simulink model "CrazyClover_thrust_angular_vel_control1"  (R2020b)
settings: Solver=VariableStepAuto  StartTime=0.0  StopTime=1.5  RelTol=1e-3
values from neighbouring files (symbols this model uses):
  controller_matrix = [mass/(4*gravity)*1000 mass/(4*gravity)*1000 mass/(4*gravity)*1000 mass/(4*gravity)*1000 ... (first row only)    [sim_param.m]
  kM1 = Armlength /sqrt(2)    [sim_param.m]
  kM2 = Armlength /sqrt(2)    [sim_param.m]
  kM3 = 1    [sim_param.m]
undefined symbols (not defined in the file or in its folder): Pitchrate, Rollrate, Yawrate
libraries: pid_lib x6
settings Model: Creator=kt012  LastModifiedBy=kt012

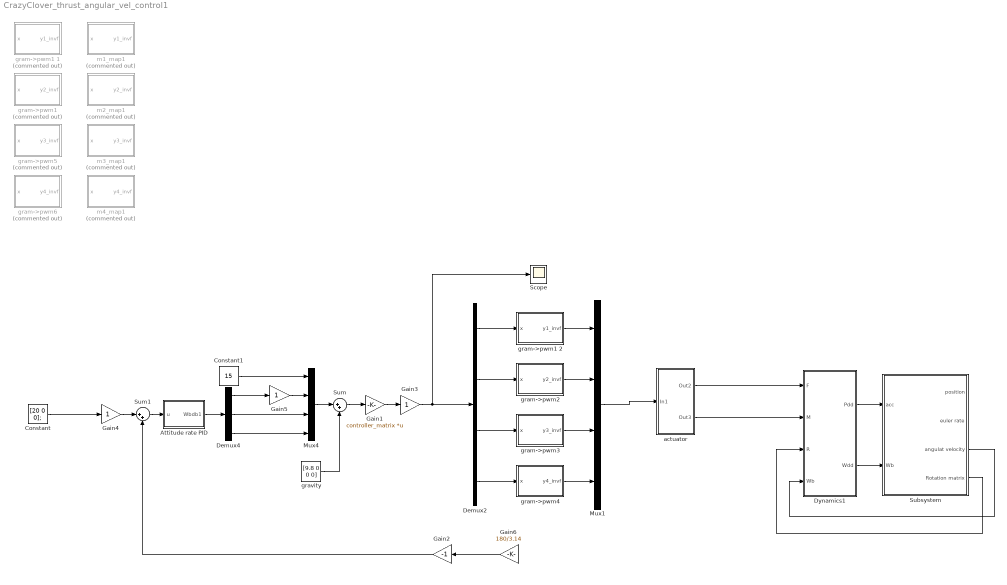
== system CrazyClover_thrust_angular_vel_control1 ==
  Attitude rate PID : Subsystem
  Constant : Constant  Value=[20 0 0];
  Constant1 : Constant  Value=15
  Demux2 : Demux
  Demux4 : Demux  Outputs=3
  Dynamics1 : MATLAB Function  TreatAsAtomicUnit=on
  Gain1 : Gain  Gain=controller_matrix  Multiplication=Matrix(K*u)
  Gain2 : Gain  Gain=-1
  Gain3 : Gain
  Gain4 : Gain
  Gain5 : Gain
  Gain6 : Gain  Gain=180/3.14
  Mux1 : Mux
  Mux4 : Mux
  Scope : Scope
  Subsystem : Subsystem
  Sum : Sum  Inputs=|++
  Sum1 : Sum  Inputs=|++
  actuator : Subsystem
  gram->pwm1 : MATLAB Function  Commented=on  TreatAsAtomicUnit=on
  gram->pwm1 1 : MATLAB Function  Commented=on  TreatAsAtomicUnit=on
  gram->pwm1 2 : MATLAB Function  TreatAsAtomicUnit=on
  gram->pwm2 : MATLAB Function  TreatAsAtomicUnit=on
  gram->pwm3 : MATLAB Function  TreatAsAtomicUnit=on
  gram->pwm4 : MATLAB Function  TreatAsAtomicUnit=on
  gram->pwm5 : MATLAB Function  Commented=on  TreatAsAtomicUnit=on
  gram->pwm6 : MATLAB Function  Commented=on  TreatAsAtomicUnit=on
  gravity : Constant  Value=[9.8 0 0 0]
  m1_map1 : MATLAB Function  Commented=on  TreatAsAtomicUnit=on
  m2_map1 : MATLAB Function  Commented=on  TreatAsAtomicUnit=on
  m3_map1 : MATLAB Function  Commented=on  TreatAsAtomicUnit=on
  m4_map1 : MATLAB Function  Commented=on  TreatAsAtomicUnit=on
  wires:
  Gain1/1 -> Gain3/1
  Gain3/1 -> Scope/1, Demux2/1
  Demux2/1 -> gram->pwm1 2/1(x)
  Demux2/2 -> gram->pwm2/1(x)
  Demux2/3 -> gram->pwm3/1(x)
  Demux2/4 -> gram->pwm4/1(x)
  gravity/1 -> Sum/2
  Sum/1 -> Gain1/1
  Attitude rate PID/1(Wbdb1) -> Demux4/1
  Gain2/1 -> Sum1/2
  Demux4/1 -> Gain5/1
  Demux4/3 -> Mux4/4
  Constant1/1 -> Mux4/1
  Mux4/1 -> Sum/1
  Demux4/2 -> Mux4/3
  Gain5/1 -> Mux4/2
  Sum1/1 -> Attitude rate PID/1(u)
  Constant/1 -> Gain4/1
  Gain4/1 -> Sum1/1
  Gain6/1 -> Gain2/1
  gram->pwm1 2/1(y1_invf) -> Mux1/1
  gram->pwm2/1(y2_invf) -> Mux1/2
  gram->pwm3/1(y3_invf) -> Mux1/3
  gram->pwm4/1(y4_invf) -> Mux1/4
  Dynamics1/1(Pdd) -> Subsystem/1(acc)
  Dynamics1/2(Wdd) -> Subsystem/2(Wb)
  Subsystem/3(angulat velocity) -> Dynamics1/4(Wb)
  Subsystem/4(Rotation matrix) -> Dynamics1/3(R)
  Mux1/1 -> actuator/1(In1)
  actuator/1(Out2) -> Dynamics1/1(F)
  actuator/2(Out3) -> Dynamics1/2(M)

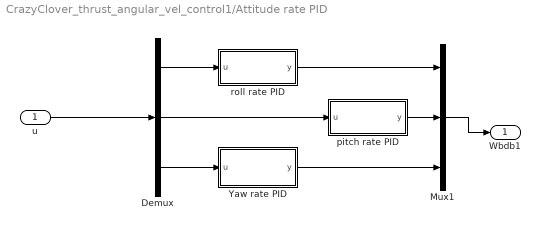
== system CrazyClover_thrust_angular_vel_control1/Attitude rate PID ==
  u : Inport
  Demux : Demux  Outputs=3
  Mux1 : Mux  Inputs=3
  "Yaw rate PID " : Subsystem
  pitch rate PID : Subsystem
  "roll rate PID " : Subsystem
  Wbdb1 : Outport
  wires:
  "roll rate PID "/1(y) -> Mux1/1
  pitch rate PID/1(y) -> Mux1/2
  Demux/2 -> pitch rate PID/1(u)
  u/1 -> Demux/1
  Demux/3 -> "Yaw rate PID "/1(u)
  Demux/1 -> "roll rate PID "/1(u)
  "Yaw rate PID "/1(y) -> Mux1/3
  Mux1/1 -> Wbdb1/1

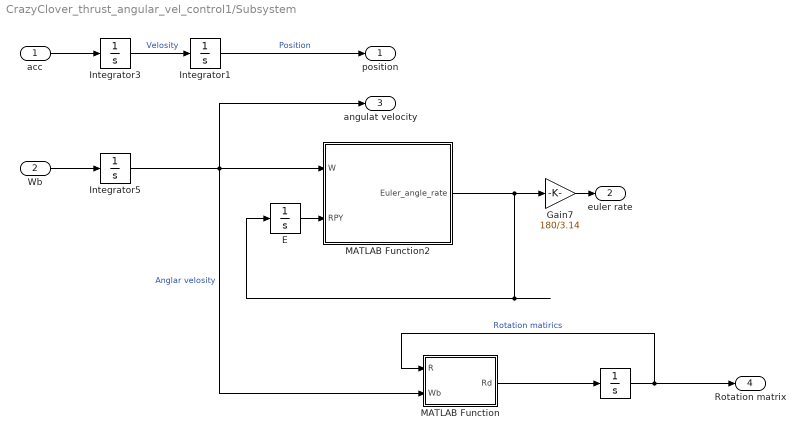
== system CrazyClover_thrust_angular_vel_control1/Subsystem ==
  acc : Inport
  Wb : Inport  Port=2
  " " : Integrator  InitialCondition=[1 0 0; 0 1 0; 0 0 1];  ContinuousStateAttributes="\"\""
  E : Integrator  InitialCondition=[0 0 0];
  Gain7 : Gain  Gain=180/3.14
  Integrator1 : Integrator  InitialCondition=[0 0 0];
  Integrator3 : Integrator  InitialCondition=[0 0 0];
  Integrator5 : Integrator  InitialCondition=[0 0 0];
  MATLAB Function : MATLAB Function  TreatAsAtomicUnit=on
  MATLAB Function2 : MATLAB Function  TreatAsAtomicUnit=on
  position : Outport
  euler rate : Outport  Port=2
  angulat velocity : Outport  Port=3
  Rotation matrix : Outport  Port=4
  wires:
  MATLAB Function2/1(Euler_angle_rate) -> E/1, Gain7/1
  acc/1 -> Integrator3/1
  Integrator1/1 -> position/1  "Position"
  Integrator3/1 -> Integrator1/1  "Velosity"
  E/1 -> MATLAB Function2/2(RPY)
  Wb/1 -> Integrator5/1
  Gain7/1 -> euler rate/1
  MATLAB Function/1(Rd) -> " "/1
  Integrator5/1 -> MATLAB Function/2(Wb), angulat velocity/1, MATLAB Function2/1(W)  "Anglar velosity"
  " "/1 -> Rotation matrix/1, MATLAB Function/1(R)  "Rotation matirics"

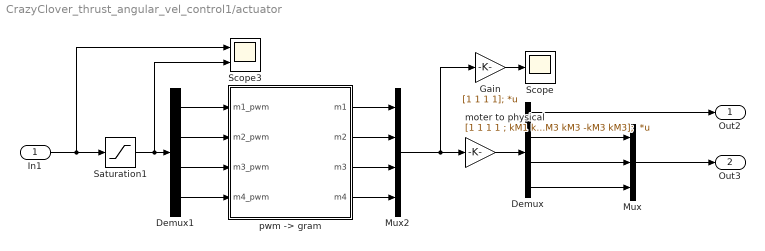
== system CrazyClover_thrust_angular_vel_control1/actuator ==
  In1 : Inport
  Demux : Demux
  Demux1 : Demux
  Gain : Gain  Gain=[1 1 1 1];  Multiplication=Matrix(K*u)
  Mux : Mux  Inputs=3
  Mux2 : Mux
  Saturation1 : Saturate  UpperLimit=40000  LowerLimit=0
  Scope : Scope
  Scope3 : Scope  NumInputPorts=2
  moter to physical : Gain  Gain=[1 1 1 1 ; kM1 kM1 -kM1 -kM1; -kM2 kM2 kM2 -kM2; -kM3 kM3 -kM3 kM3];  Multiplication=Matrix(K*u)
  "pwm -> gram" : MATLAB Function  TreatAsAtomicUnit=on
  Out2 : Outport
  Out3 : Outport  Port=2
  wires:
  Demux/2 -> Mux/1
  "pwm -> gram"/3(m3) -> Mux2/3
  Demux1/2 -> "pwm -> gram"/2(m2_pwm)
  Demux/4 -> Mux/3
  Demux/3 -> Mux/2
  moter to physical/1 -> Demux/1
  "pwm -> gram"/1(m1) -> Mux2/1
  Mux2/1 -> Gain/1, moter to physical/1
  Gain/1 -> Scope/1
  Saturation1/1 -> Scope3/2, Demux1/1
  In1/1 -> Scope3/1, Saturation1/1
  Demux1/3 -> "pwm -> gram"/3(m3_pwm)
  "pwm -> gram"/4(m4) -> Mux2/4
  "pwm -> gram"/2(m2) -> Mux2/2
  Demux1/4 -> "pwm -> gram"/4(m4_pwm)
  Demux1/1 -> "pwm -> gram"/1(m1_pwm)
  Mux/1 -> Out3/1
  Demux/1 -> Out2/1

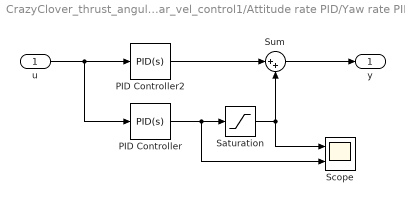
== system CrazyClover_thrust_angular_vel_control1/Attitude rate PID/Yaw rate PID  ==
  u : Inport
  PID Controller : pid_lib/PID Controller  Controller=PID  Form=Parallel  TimeDomain=Continuous-time  UseExternalTs=off  SampleTime=-1  IntegratorMethod=Forward Euler  FilterMethod=Forward Euler  ControllerParametersSource=internal  P=0  I=Yawrate.ki  D=0  UseFilter=on  N=100  TunerSelectOption=Transfer Function Based (PID Tuner App)  InitialConditionSource=internal  InitialConditionForIntegrator=0  InitialConditionForFilter=0  DifferentiatorICPrevScaledInput=0  ExternalReset=none  TrackingMode=off  Kt=1  LimitOutput=off  SatLimitsSource=internal  UpperSaturationLimit=inf  LowerSaturationLimit=-inf  LinearizeAsGain=on  AntiWindupMode=none  Kb=1  POutMin=[]  POutMax=[]  IOutMin=[]  IOutMax=[]  DOutMin=[]  DOutMax=[]  NOutMin=[]  NOutMax=[]  SumOutMin=[]  SumOutMax=[]  SaturationOutMin=[]  SaturationOutMax=[]  PParamMin=[]  PParamMax=[]  IParamMin=[]  IParamMax=[]  DParamMin=[]  DParamMax=[]  NParamMin=[]  NParamMax=[]  KbParamMin=[]  KbParamMax=[]  KtParamMin=[]  KtParamMax=[]  KbOutMin=[]  KbOutMax=[]  KtOutMin=[]  KtOutMax=[]  IntegratorOutMin=[]  IntegratorOutMax=[]  FilterOutMin=[]  FilterOutMax=[]  SumI1OutMin=[]  SumI1OutMax=[]  SumI2OutMin=[]  SumI2OutMax=[]  SumI3OutMin=[]  SumI3OutMax=[]  SumI4OutMin=[]  SumI4OutMax=[]  SumDOutMin=[]  SumDOutMax=[]  DifferentiatorOutMin=[]  DifferentiatorOutMax=[]  FilterDiffOutCoefMin=[]  FilterDiffOutCoefMax=[]  ReciprocalOutMin=[]  ReciprocalOutMax=[]  SumDenOutMin=[]  SumDenOutMax=[]  SumNumOutMin=[]  SumNumOutMax=[]  DivideOutMin=[]  DivideOutMax=[]  UdiffTsProdOutMin=[]  UdiffTsProdOutMax=[]  NTsProdOutMin=[]  NTsProdOutMax=[]  UintegralTsProdOutMin=[]  UintegralTsProdOutMax=[]  UngainTsProdOutMin=[]  UngainTsProdOutMax=[]  IntegratorContinuousStateAttributes=''  IntegratorStateMustResolveToSignalObject=off  IntegratorRTWStateStorageClass=Auto  FilterContinuousStateAttributes=''  FilterStateMustResolveToSignalObject=off  FilterRTWStateStorageClass=Auto  ParallelPVariant=InternalParameters  IdealPVariant=Disabled  IVariant=InternalParameters  DVariant=InternalParameters  IntegratorVariant=Continuous  SatVariant=Disabled  AWVariant=Passthrough  PCopyVariant=Disabled  TRVariant=Disabled  FdbkBlocksVariant=Forward  IdealPFdbkVariant=Disabled  SatFdbkVariant=Disabled  DerivativeFilterVariant=ContFilter  NVariant=InternalParameters  NCopyVariant=Disabled  FilterICVariant=InternalICsFilter  IntegratorICVariant=InternalICs  ExternalResetVariant=Disabled  TRSumVariant=Passthrough  SumFdbkVariant=Disabled  SumVariant=Sum_PID  TsampFilterVariant=InternalTs  TsampNgainVariant=Passthrough  TsampIntegralVariant=Passthrough  ExternalSaturationOutDataTypeStr=Inherit: Same as second input
  PID Controller2 : pid_lib/PID Controller  Controller=PID  Form=Parallel  TimeDomain=Continuous-time  UseExternalTs=off  SampleTime=-1  IntegratorMethod=Forward Euler  FilterMethod=Forward Euler  ControllerParametersSource=internal  P=Yawrate.kp  I=0  D=0  UseFilter=on  N=100  TunerSelectOption=Transfer Function Based (PID Tuner App)  InitialConditionSource=internal  InitialConditionForIntegrator=0  InitialConditionForFilter=0  DifferentiatorICPrevScaledInput=0  ExternalReset=none  TrackingMode=off  Kt=1  LimitOutput=off  SatLimitsSource=internal  UpperSaturationLimit=inf  LowerSaturationLimit=-inf  LinearizeAsGain=on  AntiWindupMode=none  Kb=1  POutMin=[]  POutMax=[]  IOutMin=[]  IOutMax=[]  DOutMin=[]  DOutMax=[]  NOutMin=[]  NOutMax=[]  SumOutMin=[]  SumOutMax=[]  SaturationOutMin=[]  SaturationOutMax=[]  PParamMin=[]  PParamMax=[]  IParamMin=[]  IParamMax=[]  DParamMin=[]  DParamMax=[]  NParamMin=[]  NParamMax=[]  KbParamMin=[]  KbParamMax=[]  KtParamMin=[]  KtParamMax=[]  KbOutMin=[]  KbOutMax=[]  KtOutMin=[]  KtOutMax=[]  IntegratorOutMin=[]  IntegratorOutMax=[]  FilterOutMin=[]  FilterOutMax=[]  SumI1OutMin=[]  SumI1OutMax=[]  SumI2OutMin=[]  SumI2OutMax=[]  SumI3OutMin=[]  SumI3OutMax=[]  SumI4OutMin=[]  SumI4OutMax=[]  SumDOutMin=[]  SumDOutMax=[]  DifferentiatorOutMin=[]  DifferentiatorOutMax=[]  FilterDiffOutCoefMin=[]  FilterDiffOutCoefMax=[]  ReciprocalOutMin=[]  ReciprocalOutMax=[]  SumDenOutMin=[]  SumDenOutMax=[]  SumNumOutMin=[]  SumNumOutMax=[]  DivideOutMin=[]  DivideOutMax=[]  UdiffTsProdOutMin=[]  UdiffTsProdOutMax=[]  NTsProdOutMin=[]  NTsProdOutMax=[]  UintegralTsProdOutMin=[]  UintegralTsProdOutMax=[]  UngainTsProdOutMin=[]  UngainTsProdOutMax=[]  IntegratorContinuousStateAttributes=''  IntegratorStateMustResolveToSignalObject=off  IntegratorRTWStateStorageClass=Auto  FilterContinuousStateAttributes=''  FilterStateMustResolveToSignalObject=off  FilterRTWStateStorageClass=Auto  ParallelPVariant=InternalParameters  IdealPVariant=Disabled  IVariant=InternalParameters  DVariant=InternalParameters  IntegratorVariant=Continuous  SatVariant=Disabled  AWVariant=Passthrough  PCopyVariant=Disabled  TRVariant=Disabled  FdbkBlocksVariant=Forward  IdealPFdbkVariant=Disabled  SatFdbkVariant=Disabled  DerivativeFilterVariant=ContFilter  NVariant=InternalParameters  NCopyVariant=Disabled  FilterICVariant=InternalICsFilter  IntegratorICVariant=InternalICs  ExternalResetVariant=Disabled  TRSumVariant=Passthrough  SumFdbkVariant=Disabled  SumVariant=Sum_PID  TsampFilterVariant=InternalTs  TsampNgainVariant=Passthrough  TsampIntegralVariant=Passthrough  ExternalSaturationOutDataTypeStr=Inherit: Same as second input
  Saturation : Saturate  UpperLimit=Yawrate.intupper  LowerLimit=Yawrate.intlower
  Scope : Scope  NumInputPorts=2
  Sum : Sum  Inputs=|++
  y : Outport
  wires:
  PID Controller2/1 -> Sum/1
  u/1 -> PID Controller/1, PID Controller2/1
  Sum/1 -> y/1
  PID Controller/1 -> Scope/2, Saturation/1
  Saturation/1 -> Sum/2, Scope/1

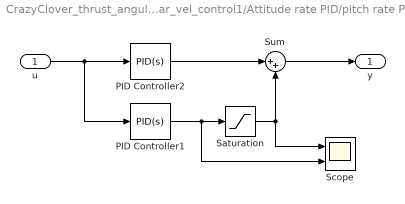
== system CrazyClover_thrust_angular_vel_control1/Attitude rate PID/pitch rate PID ==
  u : Inport
  PID Controller1 : pid_lib/PID Controller  Controller=PID  Form=Parallel  TimeDomain=Continuous-time  UseExternalTs=off  SampleTime=-1  IntegratorMethod=Forward Euler  FilterMethod=Forward Euler  ControllerParametersSource=internal  P=0  I=Pitchrate.ki  D=0  UseFilter=on  N=100  TunerSelectOption=Transfer Function Based (PID Tuner App)  InitialConditionSource=internal  InitialConditionForIntegrator=0  InitialConditionForFilter=0  DifferentiatorICPrevScaledInput=0  ExternalReset=none  TrackingMode=off  Kt=1  LimitOutput=off  SatLimitsSource=internal  UpperSaturationLimit=inf  LowerSaturationLimit=-inf  LinearizeAsGain=on  AntiWindupMode=none  Kb=1  POutMin=[]  POutMax=[]  IOutMin=[]  IOutMax=[]  DOutMin=[]  DOutMax=[]  NOutMin=[]  NOutMax=[]  SumOutMin=[]  SumOutMax=[]  SaturationOutMin=[]  SaturationOutMax=[]  PParamMin=[]  PParamMax=[]  IParamMin=[]  IParamMax=[]  DParamMin=[]  DParamMax=[]  NParamMin=[]  NParamMax=[]  KbParamMin=[]  KbParamMax=[]  KtParamMin=[]  KtParamMax=[]  KbOutMin=[]  KbOutMax=[]  KtOutMin=[]  KtOutMax=[]  IntegratorOutMin=[]  IntegratorOutMax=[]  FilterOutMin=[]  FilterOutMax=[]  SumI1OutMin=[]  SumI1OutMax=[]  SumI2OutMin=[]  SumI2OutMax=[]  SumI3OutMin=[]  SumI3OutMax=[]  SumI4OutMin=[]  SumI4OutMax=[]  SumDOutMin=[]  SumDOutMax=[]  DifferentiatorOutMin=[]  DifferentiatorOutMax=[]  FilterDiffOutCoefMin=[]  FilterDiffOutCoefMax=[]  ReciprocalOutMin=[]  ReciprocalOutMax=[]  SumDenOutMin=[]  SumDenOutMax=[]  SumNumOutMin=[]  SumNumOutMax=[]  DivideOutMin=[]  DivideOutMax=[]  UdiffTsProdOutMin=[]  UdiffTsProdOutMax=[]  NTsProdOutMin=[]  NTsProdOutMax=[]  UintegralTsProdOutMin=[]  UintegralTsProdOutMax=[]  UngainTsProdOutMin=[]  UngainTsProdOutMax=[]  IntegratorContinuousStateAttributes=''  IntegratorStateMustResolveToSignalObject=off  IntegratorRTWStateStorageClass=Auto  FilterContinuousStateAttributes=''  FilterStateMustResolveToSignalObject=off  FilterRTWStateStorageClass=Auto  ParallelPVariant=InternalParameters  IdealPVariant=Disabled  IVariant=InternalParameters  DVariant=InternalParameters  IntegratorVariant=Continuous  SatVariant=Disabled  AWVariant=Passthrough  PCopyVariant=Disabled  TRVariant=Disabled  FdbkBlocksVariant=Forward  IdealPFdbkVariant=Disabled  SatFdbkVariant=Disabled  DerivativeFilterVariant=ContFilter  NVariant=InternalParameters  NCopyVariant=Disabled  FilterICVariant=InternalICsFilter  IntegratorICVariant=InternalICs  ExternalResetVariant=Disabled  TRSumVariant=Passthrough  SumFdbkVariant=Disabled  SumVariant=Sum_PID  TsampFilterVariant=InternalTs  TsampNgainVariant=Passthrough  TsampIntegralVariant=Passthrough  ExternalSaturationOutDataTypeStr=Inherit: Same as second input
  PID Controller2 : pid_lib/PID Controller  Controller=PID  Form=Parallel  TimeDomain=Continuous-time  UseExternalTs=off  SampleTime=-1  IntegratorMethod=Forward Euler  FilterMethod=Forward Euler  ControllerParametersSource=internal  P=Pitchrate.kp  I=0  D=0  UseFilter=on  N=100  TunerSelectOption=Transfer Function Based (PID Tuner App)  InitialConditionSource=internal  InitialConditionForIntegrator=0  InitialConditionForFilter=0  DifferentiatorICPrevScaledInput=0  ExternalReset=none  TrackingMode=off  Kt=1  LimitOutput=off  SatLimitsSource=internal  UpperSaturationLimit=inf  LowerSaturationLimit=-inf  LinearizeAsGain=on  AntiWindupMode=none  Kb=1  POutMin=[]  POutMax=[]  IOutMin=[]  IOutMax=[]  DOutMin=[]  DOutMax=[]  NOutMin=[]  NOutMax=[]  SumOutMin=[]  SumOutMax=[]  SaturationOutMin=[]  SaturationOutMax=[]  PParamMin=[]  PParamMax=[]  IParamMin=[]  IParamMax=[]  DParamMin=[]  DParamMax=[]  NParamMin=[]  NParamMax=[]  KbParamMin=[]  KbParamMax=[]  KtParamMin=[]  KtParamMax=[]  KbOutMin=[]  KbOutMax=[]  KtOutMin=[]  KtOutMax=[]  IntegratorOutMin=[]  IntegratorOutMax=[]  FilterOutMin=[]  FilterOutMax=[]  SumI1OutMin=[]  SumI1OutMax=[]  SumI2OutMin=[]  SumI2OutMax=[]  SumI3OutMin=[]  SumI3OutMax=[]  SumI4OutMin=[]  SumI4OutMax=[]  SumDOutMin=[]  SumDOutMax=[]  DifferentiatorOutMin=[]  DifferentiatorOutMax=[]  FilterDiffOutCoefMin=[]  FilterDiffOutCoefMax=[]  ReciprocalOutMin=[]  ReciprocalOutMax=[]  SumDenOutMin=[]  SumDenOutMax=[]  SumNumOutMin=[]  SumNumOutMax=[]  DivideOutMin=[]  DivideOutMax=[]  UdiffTsProdOutMin=[]  UdiffTsProdOutMax=[]  NTsProdOutMin=[]  NTsProdOutMax=[]  UintegralTsProdOutMin=[]  UintegralTsProdOutMax=[]  UngainTsProdOutMin=[]  UngainTsProdOutMax=[]  IntegratorContinuousStateAttributes=''  IntegratorStateMustResolveToSignalObject=off  IntegratorRTWStateStorageClass=Auto  FilterContinuousStateAttributes=''  FilterStateMustResolveToSignalObject=off  FilterRTWStateStorageClass=Auto  ParallelPVariant=InternalParameters  IdealPVariant=Disabled  IVariant=InternalParameters  DVariant=InternalParameters  IntegratorVariant=Continuous  SatVariant=Disabled  AWVariant=Passthrough  PCopyVariant=Disabled  TRVariant=Disabled  FdbkBlocksVariant=Forward  IdealPFdbkVariant=Disabled  SatFdbkVariant=Disabled  DerivativeFilterVariant=ContFilter  NVariant=InternalParameters  NCopyVariant=Disabled  FilterICVariant=InternalICsFilter  IntegratorICVariant=InternalICs  ExternalResetVariant=Disabled  TRSumVariant=Passthrough  SumFdbkVariant=Disabled  SumVariant=Sum_PID  TsampFilterVariant=InternalTs  TsampNgainVariant=Passthrough  TsampIntegralVariant=Passthrough  ExternalSaturationOutDataTypeStr=Inherit: Same as second input
  Saturation : Saturate  UpperLimit=Pitchrate.intupper  LowerLimit=Pitchrate.intlower
  Scope : Scope  NumInputPorts=2
  Sum : Sum  Inputs=|++
  y : Outport
  wires:
  PID Controller2/1 -> Sum/1
  u/1 -> PID Controller1/1, PID Controller2/1
  Sum/1 -> y/1
  PID Controller1/1 -> Scope/2, Saturation/1
  Saturation/1 -> Sum/2, Scope/1

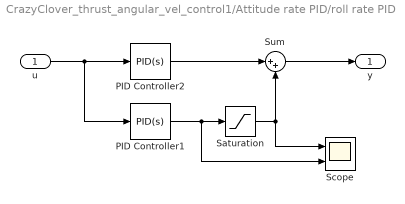
== system CrazyClover_thrust_angular_vel_control1/Attitude rate PID/roll rate PID  ==
  u : Inport
  PID Controller1 : pid_lib/PID Controller  Controller=PID  Form=Parallel  TimeDomain=Continuous-time  UseExternalTs=off  SampleTime=-1  IntegratorMethod=Forward Euler  FilterMethod=Forward Euler  ControllerParametersSource=internal  P=0  I=Rollrate.ki  D=0  UseFilter=on  N=100  TunerSelectOption=Transfer Function Based (PID Tuner App)  InitialConditionSource=internal  InitialConditionForIntegrator=0  InitialConditionForFilter=0  DifferentiatorICPrevScaledInput=0  ExternalReset=none  TrackingMode=off  Kt=1  LimitOutput=off  SatLimitsSource=internal  UpperSaturationLimit=inf  LowerSaturationLimit=-inf  LinearizeAsGain=on  AntiWindupMode=none  Kb=1  POutMin=[]  POutMax=[]  IOutMin=[]  IOutMax=[]  DOutMin=[]  DOutMax=[]  NOutMin=[]  NOutMax=[]  SumOutMin=[]  SumOutMax=[]  SaturationOutMin=[]  SaturationOutMax=[]  PParamMin=[]  PParamMax=[]  IParamMin=[]  IParamMax=[]  DParamMin=[]  DParamMax=[]  NParamMin=[]  NParamMax=[]  KbParamMin=[]  KbParamMax=[]  KtParamMin=[]  KtParamMax=[]  KbOutMin=[]  KbOutMax=[]  KtOutMin=[]  KtOutMax=[]  IntegratorOutMin=[]  IntegratorOutMax=[]  FilterOutMin=[]  FilterOutMax=[]  SumI1OutMin=[]  SumI1OutMax=[]  SumI2OutMin=[]  SumI2OutMax=[]  SumI3OutMin=[]  SumI3OutMax=[]  SumI4OutMin=[]  SumI4OutMax=[]  SumDOutMin=[]  SumDOutMax=[]  DifferentiatorOutMin=[]  DifferentiatorOutMax=[]  FilterDiffOutCoefMin=[]  FilterDiffOutCoefMax=[]  ReciprocalOutMin=[]  ReciprocalOutMax=[]  SumDenOutMin=[]  SumDenOutMax=[]  SumNumOutMin=[]  SumNumOutMax=[]  DivideOutMin=[]  DivideOutMax=[]  UdiffTsProdOutMin=[]  UdiffTsProdOutMax=[]  NTsProdOutMin=[]  NTsProdOutMax=[]  UintegralTsProdOutMin=[]  UintegralTsProdOutMax=[]  UngainTsProdOutMin=[]  UngainTsProdOutMax=[]  IntegratorContinuousStateAttributes=''  IntegratorStateMustResolveToSignalObject=off  IntegratorRTWStateStorageClass=Auto  FilterContinuousStateAttributes=''  FilterStateMustResolveToSignalObject=off  FilterRTWStateStorageClass=Auto  ParallelPVariant=InternalParameters  IdealPVariant=Disabled  IVariant=InternalParameters  DVariant=InternalParameters  IntegratorVariant=Continuous  SatVariant=Disabled  AWVariant=Passthrough  PCopyVariant=Disabled  TRVariant=Disabled  FdbkBlocksVariant=Forward  IdealPFdbkVariant=Disabled  SatFdbkVariant=Disabled  DerivativeFilterVariant=ContFilter  NVariant=InternalParameters  NCopyVariant=Disabled  FilterICVariant=InternalICsFilter  IntegratorICVariant=InternalICs  ExternalResetVariant=Disabled  TRSumVariant=Passthrough  SumFdbkVariant=Disabled  SumVariant=Sum_PID  TsampFilterVariant=InternalTs  TsampNgainVariant=Passthrough  TsampIntegralVariant=Passthrough  ExternalSaturationOutDataTypeStr=Inherit: Same as second input
  PID Controller2 : pid_lib/PID Controller  Controller=PID  Form=Parallel  TimeDomain=Continuous-time  UseExternalTs=off  SampleTime=-1  IntegratorMethod=Forward Euler  FilterMethod=Forward Euler  ControllerParametersSource=internal  P=Rollrate.kp  I=0  D=0  UseFilter=on  N=100  TunerSelectOption=Transfer Function Based (PID Tuner App)  InitialConditionSource=internal  InitialConditionForIntegrator=0  InitialConditionForFilter=0  DifferentiatorICPrevScaledInput=0  ExternalReset=none  TrackingMode=off  Kt=1  LimitOutput=off  SatLimitsSource=internal  UpperSaturationLimit=inf  LowerSaturationLimit=-inf  LinearizeAsGain=on  AntiWindupMode=none  Kb=1  POutMin=[]  POutMax=[]  IOutMin=[]  IOutMax=[]  DOutMin=[]  DOutMax=[]  NOutMin=[]  NOutMax=[]  SumOutMin=[]  SumOutMax=[]  SaturationOutMin=[]  SaturationOutMax=[]  PParamMin=[]  PParamMax=[]  IParamMin=[]  IParamMax=[]  DParamMin=[]  DParamMax=[]  NParamMin=[]  NParamMax=[]  KbParamMin=[]  KbParamMax=[]  KtParamMin=[]  KtParamMax=[]  KbOutMin=[]  KbOutMax=[]  KtOutMin=[]  KtOutMax=[]  IntegratorOutMin=[]  IntegratorOutMax=[]  FilterOutMin=[]  FilterOutMax=[]  SumI1OutMin=[]  SumI1OutMax=[]  SumI2OutMin=[]  SumI2OutMax=[]  SumI3OutMin=[]  SumI3OutMax=[]  SumI4OutMin=[]  SumI4OutMax=[]  SumDOutMin=[]  SumDOutMax=[]  DifferentiatorOutMin=[]  DifferentiatorOutMax=[]  FilterDiffOutCoefMin=[]  FilterDiffOutCoefMax=[]  ReciprocalOutMin=[]  ReciprocalOutMax=[]  SumDenOutMin=[]  SumDenOutMax=[]  SumNumOutMin=[]  SumNumOutMax=[]  DivideOutMin=[]  DivideOutMax=[]  UdiffTsProdOutMin=[]  UdiffTsProdOutMax=[]  NTsProdOutMin=[]  NTsProdOutMax=[]  UintegralTsProdOutMin=[]  UintegralTsProdOutMax=[]  UngainTsProdOutMin=[]  UngainTsProdOutMax=[]  IntegratorContinuousStateAttributes=''  IntegratorStateMustResolveToSignalObject=off  IntegratorRTWStateStorageClass=Auto  FilterContinuousStateAttributes=''  FilterStateMustResolveToSignalObject=off  FilterRTWStateStorageClass=Auto  ParallelPVariant=InternalParameters  IdealPVariant=Disabled  IVariant=InternalParameters  DVariant=InternalParameters  IntegratorVariant=Continuous  SatVariant=Disabled  AWVariant=Passthrough  PCopyVariant=Disabled  TRVariant=Disabled  FdbkBlocksVariant=Forward  IdealPFdbkVariant=Disabled  SatFdbkVariant=Disabled  DerivativeFilterVariant=ContFilter  NVariant=InternalParameters  NCopyVariant=Disabled  FilterICVariant=InternalICsFilter  IntegratorICVariant=InternalICs  ExternalResetVariant=Disabled  TRSumVariant=Passthrough  SumFdbkVariant=Disabled  SumVariant=Sum_PID  TsampFilterVariant=InternalTs  TsampNgainVariant=Passthrough  TsampIntegralVariant=Passthrough  ExternalSaturationOutDataTypeStr=Inherit: Same as second input
  Saturation : Saturate  UpperLimit=Rollrate.intupper  LowerLimit=Rollrate.intlower
  Scope : Scope  NumInputPorts=2
  Sum : Sum  Inputs=|++
  y : Outport
  wires:
  Saturation/1 -> Scope/1, Sum/2
  PID Controller1/1 -> Saturation/1, Scope/2
  Sum/1 -> y/1
  u/1 -> PID Controller2/1, PID Controller1/1
  PID Controller2/1 -> Sum/1

== matlab function CrazyClover_thrust_angular_vel_control1/gram->pwm2 ==
  data: x input; y2_invf output
function y2_invf = m2_map(x)
%#codegen

%    This function was generated by the Symbolic Math Toolbox version 8.6.
%    24-Aug-2022 00:51:31
if x > 0
    y2_invf = sqrt(x.*8.763965396891775e-7+1.033956593757182e-5).*2.282071995297151e+6-5.020028004430765e+3;
else
    x = abs(x);
    y2_invf = -(sqrt(x.*8.763965396891775e-7+1.033956593757182e-5).*2.282071995297151e+6-5.020028004430765e+3);
end

== matlab function CrazyClover_thrust_angular_vel_control1/gram->pwm3 ==
  data: x input; y3_invf output
function y3_invf = m3_map(x)
%#codegen

%    This function was generated by the Symbolic Math Toolbox version 8.6.
%    24-Aug-2022 00:51:31

if x > 0
    y3_invf = sqrt(x.*8.464410710967024e-7+1.206468234853723e-5).*2.362834305061159e+6-5.75446231128539e+3;
else
    x = abs(x);
    y3_invf = -(sqrt(x.*8.464410710967024e-7+1.206468234853723e-5).*2.362834305061159e+6-5.75446231128539e+3);
end

== matlab function CrazyClover_thrust_angular_vel_control1/gram->pwm4 ==
  data: x input; y4_invf output
function y4_invf = m4_map(x)
%#codegen

%    This function was generated by the Symbolic Math Toolbox version 8.6.
%    24-Aug-2022 00:51:31
if x > 0
    y4_invf = sqrt(x.*8.083914057959226e-7+1.102319411174238e-5).*2.474049062942287e+6-5.961111523577613e+3;
else
    x = abs(x);
    y4_invf = -(sqrt(x.*8.083914057959226e-7+1.102319411174238e-5).*2.474049062942287e+6-5.961111523577613e+3);
end

== matlab function CrazyClover_thrust_angular_vel_control1/gram->pwm1 ==
  data: x input; y2_invf output
function y2_invf = m2_map(x)
%#codegen

%    This function was generated by the Symbolic Math Toolbox version 8.6.
%    24-Aug-2022 00:51:31
if x > 0
    y2_invf = sqrt(x.*8.763965396891775e-7+1.033956593757182e-5).*2.282071995297151e+6-5.020028004430765e+3;
else
    x = abs(x);
    y2_invf = -(sqrt(x.*8.763965396891775e-7+1.033956593757182e-5).*2.282071995297151e+6-5.020028004430765e+3);
end

== matlab function CrazyClover_thrust_angular_vel_control1/gram->pwm1 1 ==
  data: x input; y1_invf output
function y1_invf = m1_map(x)
%#codegen

%    This function was generated by the Symbolic Math Toolbox version 8.6.
%    24-Aug-2022 00:51:31
if x > 0
    y1_invf = sqrt(x.*8.309953163553529e-7+8.77420076969215e-6).*2.406752433662037e+6-4.951128620134714e+3;
else
    x = abs(x);
    y1_invf = -(sqrt(x.*8.309953163553529e-7+8.77420076969215e-6).*2.406752433662037e+6-4.951128620134714e+3);
end

== matlab function CrazyClover_thrust_angular_vel_control1/gram->pwm5 ==
  data: x input; y3_invf output
function y3_invf = m3_map(x)
%#codegen

%    This function was generated by the Symbolic Math Toolbox version 8.6.
%    24-Aug-2022 00:51:31

if x > 0
    y3_invf = sqrt(x.*8.464410710967024e-7+1.206468234853723e-5).*2.362834305061159e+6-5.75446231128539e+3;
else
    x = abs(x);
    y3_invf = -(sqrt(x.*8.464410710967024e-7+1.206468234853723e-5).*2.362834305061159e+6-5.75446231128539e+3);
end

== matlab function CrazyClover_thrust_angular_vel_control1/gram->pwm6 ==
  data: x input; y4_invf output
function y4_invf = m4_map(x)
%#codegen

%    This function was generated by the Symbolic Math Toolbox version 8.6.
%    24-Aug-2022 00:51:31
if x > 0
    y4_invf = sqrt(x.*8.083914057959226e-7+1.102319411174238e-5).*2.474049062942287e+6-5.961111523577613e+3;
else
    x = abs(x);
    y4_invf = -(sqrt(x.*8.083914057959226e-7+1.102319411174238e-5).*2.474049062942287e+6-5.961111523577613e+3);
end

== matlab function CrazyClover_thrust_angular_vel_control1/Subsystem/MATLAB Function ==
  data: R input; Rd output; Wb input
function Rd = fcn(R, Wb)
wx = Wb(1);
wy = Wb(2);
wz = Wb(3);
Wb = [ 0    -wz   wy;
       wz    0   -wx;
      -wy    wx   0];
Rd = R * Wb;

== matlab function CrazyClover_thrust_angular_vel_control1/m1_map1 ==
  data: x input; y1_invf output
function y1_invf = m1_map(x)
%#codegen

%    This function was generated by the Symbolic Math Toolbox version 8.6.
%    24-Aug-2022 01:21:23

y1_invf = sqrt(x.*8.309953163553529e-7+8.77420076969215e-6).*2.406752433662037e+6-4.951128620134714e+3;

== matlab function CrazyClover_thrust_angular_vel_control1/m2_map1 ==
  data: x input; y2_invf output
function y2_invf = m2_map(x)
%#codegen

%    This function was generated by the Symbolic Math Toolbox version 8.6.
%    24-Aug-2022 01:21:23

y2_invf = sqrt(x.*8.763965396891775e-7+1.033956593757182e-5).*2.282071995297151e+6-5.020028004430765e+3;

== matlab function CrazyClover_thrust_angular_vel_control1/m3_map1 ==
  data: x input; y3_invf output
function y3_invf = m3_map(x)
%#codegen

%    This function was generated by the Symbolic Math Toolbox version 8.6.
%    24-Aug-2022 01:21:23

y3_invf = sqrt(x.*8.464410710967024e-7+1.206468234853723e-5).*2.362834305061159e+6-5.75446231128539e+3;

== matlab function CrazyClover_thrust_angular_vel_control1/actuator/pwm -> gram ==
  data: m1_pwm input; m1 output; m2_pwm input; m3_pwm input; m4_pwm input; m2 output; m3 output; m4 output
function [m1, m2,m3, m4]= func(m1_pwm, m2_pwm, m3_pwm, m4_pwm)

% F [16bit] Wddb [16bit]

% m1_pwm = moter_in(1);
% m2_pwm = moter_in(2);
% m3_pwm = moter_in(3);
% m4_pwm = moter_in(4);
m1_map = [2.1910e-07 0.0022 0];
m2_map = [2.1910e-07 0.0022 0];
m3_map = [2.1161e-07 0.0024 0];
m4_map = [2.0210e-07 0.0024 0];
% m_avs = (m1_pwm + m2_pwm + m3_pwm + m4_pwm)/4;
% m1_pwm = m_avs;
% m2_pwm = m_avs;
% m3_pwm = m_avs;
% m4_pwm = m_avs;
if m1_pwm > 0
    m1 = m1_map * [m1_pwm^2;m1_pwm;1];
else
    m1 = -m1_map * [m1_pwm^2;-m1_pwm;1];
end
if m2_pwm > 0
    m2 = m2_map * [m2_pwm^2;m2_pwm;1];
else
    m2 = -m2_map * [m2_pwm^2;-m2_pwm;1];
end
if m3_pwm > 0
    m3 = m3_map * [m3_pwm^2;m3_pwm;1];
else
    m3 = -m3_map * [m3_pwm^2;-m3_pwm;1];
end
if m1_pwm > 0
    m4 = m4_map * [m4_pwm^2;m4_pwm;1];
else
    m4 = -m4_map * [m4_pwm^2;-m4_pwm;1];
end

== matlab function CrazyClover_thrust_angular_vel_control1/m4_map1 ==
  data: x input; y4_invf output
function y4_invf = m4_map(x)
%#codegen

%    This function was generated by the Symbolic Math Toolbox version 8.6.
%    24-Aug-2022 01:21:23

y4_invf = sqrt(x.*8.083914057959226e-7+1.102319411174238e-5).*2.474049062942287e+6-5.961111523577613e+3;

== matlab function CrazyClover_thrust_angular_vel_control1/Subsystem/MATLAB Function2 ==
  data: W input; Euler_angle_rate output; RPY input
function Euler_angle_rate = fcn(W, RPY)
roll = RPY(1);
pitch = RPY(2);
yaw = RPY(3);
rollS = sin(roll); rollC = cos(roll);           
pitchS = sin(pitch); pitchC = cos(pitch);       


Euler_angle_rate = pinv([1 0 -pitchS;
     0 rollC  pitchC * rollS;
     0 -rollS pitchC * rollC]) * W;

== matlab function CrazyClover_thrust_angular_vel_control1/gram->pwm1 2 ==
  data: x input; y1_invf output
function y1_invf = m1_map(x)
%#codegen

%    This function was generated by the Symbolic Math Toolbox version 8.6.
%    24-Aug-2022 00:51:31
if x > 0
    y1_invf = sqrt(x.*8.309953163553529e-7+8.77420076969215e-6).*2.406752433662037e+6-4.951128620134714e+3;
else
    x = abs(x);
    y1_invf = -(sqrt(x.*8.309953163553529e-7+8.77420076969215e-6).*2.406752433662037e+6-4.951128620134714e+3);
end

== matlab function CrazyClover_thrust_angular_vel_control1/Dynamics1 ==
  data: F input; Pdd output; M input; R input; Wb input; Wdd output
function [Pdd, Wdd]  = fcn(F, M, R, Wb)
m = 500;
e3 = [0 0 1]';
g = 9.8;

% 各加速度計算（ボディー座標系）
Pdd = 9.8 * F*R*e3/m - g*e3;
I = [1 0 0;
     0 1 0;
     0 0 1]*10^(-3);
% 各加速度計算（ボディー座標系）
Wdd = pinv(I)*(M - cross(Wb, I * Wb));
